simulink model "Project_Trial2"  (R2021a)
settings: Solver=VariableStepAuto  StartTime=0.0  StopTime=10.0  RelTol=1e-3
values from neighbouring files (symbols this model uses):
  X = input(Prompt)    [Project_Trial2_Run.m]
settings Model: Creator=muzaf  LastModifiedBy=muzaf

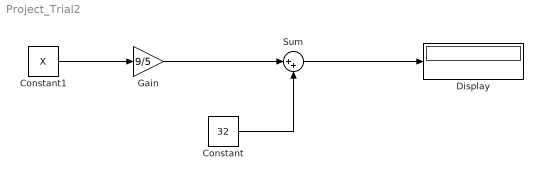
== system Project_Trial2 ==
  Constant : Constant  Value=32
  Constant1 : Constant  Value=X
  Display : Display
  Gain : Gain  Gain=9/5
  Sum : Sum  Inputs=|++
  wires:
  Constant/1 -> Sum/2
  Gain/1 -> Sum/1
  Sum/1 -> Display/1
  Constant1/1 -> Gain/1
